simulink model "simulation"  (R2024b)
settings: Solver=ode45  StartTime=0.0  StopTime=10  MaxStep=0.001  RelTol=1e-2  AbsTol=1e-2  EnableMultiTasking=on
values from neighbouring files (symbols this model uses):
  m = subs(obj.M, [obj.theta0, obj.theta1, obj.theta2, obj.L], [a0, a1, a2, l])    [VMC_test.m]
  N = m_p*(x_ddot+L*theta_ddot*cos(theta)-L*theta_dot^2*sin(theta))+N_M    [LQR_wang.m]    (also in untitled.m = length(t))
  X = [x,x_dot,phi,phi_dot,theta,theta_dot].'    [LQR_wang.m]    (also in init.m = [x, d_x, phi, d_phi, theta, d_theta].'; raw.m = [x, d_x, phi, d_phi, theta, d_theta].')
undefined symbols (not defined in the file or in its folder): big_rod, little_rod, load, main_body, MO_L, motor, wheel, Y, Z
libraries: sm_lib x92, nesl_utility x49, slpidlib x2
(part 1 of 3)
settings Model: Creator=Orwell  LastModifiedBy=Orwell
settings SolverCC: AlgebraicLoopSolver=TrustRegion  MaxZcPerStep=1
settings DataIOCC: LimitDataPoints=on  MaxDataPoints=10000  ReturnWorkspaceOutputs=off
settings OptimizationCC: ReuseModelBlockBuffer=off  LifeSpan=inf
settings DebuggingCC: UnconnectedInputMsg=warning  UnconnectedOutputMsg=warning  UnconnectedLineMsg=warning  AllowSymbolicDim=off  SubsystemReferenceDiagnosticForUnitTest=warning  SFUnexpectedBacktrackingDiag=warning  SFNoUnconditionalDefaultTransitionDiag=warning  SFExecutionAtInitializationDiag=none  ArithmeticOperatorsInVariantConditions=warning
settings ModelReferenceCC: EnableRefExpFcnMdlSchedulingChecks=on
settings SFSimCC: SimUseLocalCustomCode=off  CustomCodeUndefinedFunction=UseInterfaceOnly
settings RTWCC: RTWUseLocalCustomCode=off  GPUComputeCapability=3.5  DLArmComputeVersion=19.05
settings CodeAppCC: StateflowObjectComments=on
settings GRTTargetCC: TargetLangStandard=C89/C90 (ANSI)
settings ConfigComp: CovMetricSettings=dw  CovSaveCumulativeToWorkspaceVar=on  CovSaveSingleToWorkspaceVar=on  CovExternalEMLEnable=off  CovSFcnEnable=off
settings SimscapeCC: SimscapeLogType=all  SimscapeLogSimulationStatistics=on  SimscapeLogDataHistory=10000

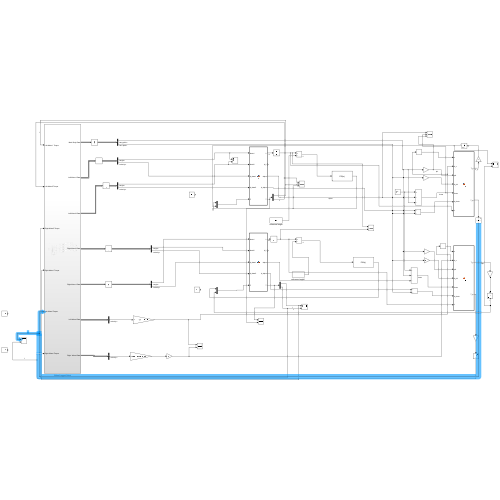
[thumbnail: Simulink's stored preview of the top-level diagram]
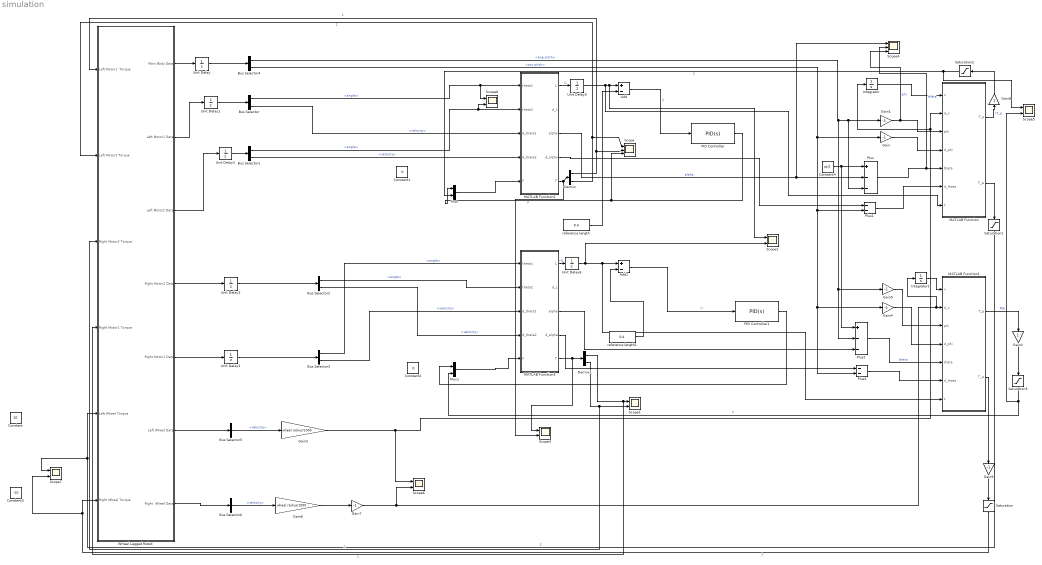
== system simulation ==
  Add : Sum  Inputs=+-
  Add1 : Sum  Inputs=+-
  Bus Selector{,1..3} (4 alike) : BusSelector  OutputSignals=angle,velocity
  Bus Selector4 : BusSelector  OutputSignals=ang pitch,acc pitch
  Bus Selector5 : BusSelector  OutputSignals=velocity
  Bus Selector6 : BusSelector  OutputSignals=velocity
  Constant : Constant  Value=10
  Constant1 : Constant  Value=0
  Constant2 : Constant  Value=0
  Constant3 : Constant  Value=-10
  Constant4 : Constant  Value=pi/2
  Demux : Demux  Outputs=2
  Demux1 : Demux  Outputs=2
  Gain{,1,4..5,7,9} (6 alike) : Gain  Gain=-1
  Gain2 : Gain  Gain=wheel.radius/1000
  Gain3 : Gain
  Gain6 : Gain  Gain=wheel.radius/1000
  Gain8 : Gain
  Integrator : Integrator
  Integrator1 : Integrator
  MATLAB Function : MATLAB Function  TreatAsAtomicUnit=on
  MATLAB Function1 : MATLAB Function  TreatAsAtomicUnit=on
  MATLAB Function2 : MATLAB Function  TreatAsAtomicUnit=on
  MATLAB Function3 : MATLAB Function  TreatAsAtomicUnit=on
  Mux : Mux  Inputs=2
  Mux1 : Mux  Inputs=2
  PID Controller : slpidlib/PID Controller  Controller=PID  Form=Parallel  TimeDomain=Continuous-time  UseExternalTs=off  SampleTime=-1  IntegratorMethod=Forward Euler  FilterMethod=Forward Euler  ControllerParametersSource=internal  P=2000  I=0  UseKiTs=off  D=0  UseExternalDerivativeSource=off  N=100  UseFilter=on  TunerSelectOption=Transfer Function Based (PID Tuner App)  InitialConditionSource=internal  InitialConditionForIntegrator=0  InitialConditionForFilter=0  DifferentiatorICPrevScaledInput=0  ExternalReset=none  TrackingMode=off  Kt=1  LimitOutput=off  SatLimitsSource=internal  UpperSaturationLimit=inf  LowerSaturationLimit=-inf  LinearizeAsGain=on  AntiWindupMode=none  Kb=1  LimitIntegrator=off  UpperIntegratorSaturationLimit=inf  LowerIntegratorSaturationLimit=-inf  POutMin=[]  POutMax=[]  IOutMin=[]  IOutMax=[]  DOutMin=[]  DOutMax=[]  NOutMin=[]  NOutMax=[]  SumOutMin=[]  SumOutMax=[]  SaturationOutMin=[]  SaturationOutMax=[]  PParamMin=[]  PParamMax=[]  IParamMin=[]  IParamMax=[]  DParamMin=[]  DParamMax=[]  NParamMin=[]  NParamMax=[]  KbParamMin=[]  KbParamMax=[]  KtParamMin=[]  KtParamMax=[]  KbOutMin=[]  KbOutMax=[]  KtOutMin=[]  KtOutMax=[]  IntegratorOutMin=[]  IntegratorOutMax=[]  FilterOutMin=[]  FilterOutMax=[]  SumI1OutMin=[]  SumI1OutMax=[]  SumI2OutMin=[]  SumI2OutMax=[]  SumI3OutMin=[]  SumI3OutMax=[]  SumI4OutMin=[]  SumI4OutMax=[]  SumDOutMin=[]  SumDOutMax=[]  DifferentiatorOutMin=[]  DifferentiatorOutMax=[]  FilterDiffOutCoefMin=[]  FilterDiffOutCoefMax=[]  ReciprocalOutMin=[]  ReciprocalOutMax=[]  SumDenOutMin=[]  SumDenOutMax=[]  SumNumOutMin=[]  SumNumOutMax=[]  DivideOutMin=[]  DivideOutMax=[]  UdiffTsProdOutMin=[]  UdiffTsProdOutMax=[]  NTsProdOutMin=[]  NTsProdOutMax=[]  UintegralTsProdOutMin=[]  UintegralTsProdOutMax=[]  UngainTsProdOutMin=[]  UngainTsProdOutMax=[]  ClampingZeroOutDataTypeStr=Inherit: Inherit via back propagation  ClampingZeroOutMin=[]  ClampingZeroOutMax=[]  FilterDenConstantOutDataTypeStr=Inherit: Inherit via back propagation  FilterDenConstantOutMin=[]  FilterDenConstantOutMax=[]  PCopyOutDataTypeStr=Inherit: Inherit via back propagation  PCopyOutMin=[]  PCopyOutMax=[]  NCopyOutDataTypeStr=Inherit: Inherit via back propagation  NCopyOutMin=[]  NCopyOutMax=[]  IntegratorContinuousStateAttributes=''  IntegratorStateMustResolveToSignalObject=off  IntegratorRTWStateStorageClass=Auto  FilterContinuousStateAttributes=''  FilterStateMustResolveToSignalObject=off  FilterRTWStateStorageClass=Auto  ParallelPVariant=InternalParameters  IdealPVariant=Disabled  IVariant=InternalParameters  DVariant=InternalParameters  IntegratorVariant=Continuous  SatVariant=Disabled  AWVariant=Passthrough  PCopyVariant=Disabled  TRVariant=Disabled  FdbkBlocksVariant=Forward  IdealPFdbkVariant=Disabled  SatFdbkVariant=Disabled  DerivativeFilterVariant=ContFilter  NVariant=InternalParameters  NCopyVariant=Disabled  FilterICVariant=InternalICsFilter  IntegratorICVariant=InternalICs  ExternalResetVariant=Disabled  TRSumVariant=Passthrough  SumFdbkVariant=Disabled  SumVariant=Sum_PID  TsampFilterVariant=InternalTs  TsampNgainVariant=Passthrough  TsampIntegralVariant=Disabled_SignalSpec  ExternalSaturationOutDataTypeStr=Inherit: Same as second input  DerivativeSourceVariant=ErrorSignal  PreIntVariant=InternalPreInt
  PID Controller1 : slpidlib/PID Controller  Controller=PID  Form=Parallel  TimeDomain=Continuous-time  UseExternalTs=off  SampleTime=-1  IntegratorMethod=Forward Euler  FilterMethod=Forward Euler  ControllerParametersSource=internal  P=2000  I=0  UseKiTs=off  D=0  UseExternalDerivativeSource=off  N=100  UseFilter=on  TunerSelectOption=Transfer Function Based (PID Tuner App)  InitialConditionSource=internal  InitialConditionForIntegrator=0  InitialConditionForFilter=0  DifferentiatorICPrevScaledInput=0  ExternalReset=none  TrackingMode=off  Kt=1  LimitOutput=off  SatLimitsSource=internal  UpperSaturationLimit=inf  LowerSaturationLimit=-inf  LinearizeAsGain=on  AntiWindupMode=none  Kb=1  LimitIntegrator=off  UpperIntegratorSaturationLimit=inf  LowerIntegratorSaturationLimit=-inf  POutMin=[]  POutMax=[]  IOutMin=[]  IOutMax=[]  DOutMin=[]  DOutMax=[]  NOutMin=[]  NOutMax=[]  SumOutMin=[]  SumOutMax=[]  SaturationOutMin=[]  SaturationOutMax=[]  PParamMin=[]  PParamMax=[]  IParamMin=[]  IParamMax=[]  DParamMin=[]  DParamMax=[]  NParamMin=[]  NParamMax=[]  KbParamMin=[]  KbParamMax=[]  KtParamMin=[]  KtParamMax=[]  KbOutMin=[]  KbOutMax=[]  KtOutMin=[]  KtOutMax=[]  IntegratorOutMin=[]  IntegratorOutMax=[]  FilterOutMin=[]  FilterOutMax=[]  SumI1OutMin=[]  SumI1OutMax=[]  SumI2OutMin=[]  SumI2OutMax=[]  SumI3OutMin=[]  SumI3OutMax=[]  SumI4OutMin=[]  SumI4OutMax=[]  SumDOutMin=[]  SumDOutMax=[]  DifferentiatorOutMin=[]  DifferentiatorOutMax=[]  FilterDiffOutCoefMin=[]  FilterDiffOutCoefMax=[]  ReciprocalOutMin=[]  ReciprocalOutMax=[]  SumDenOutMin=[]  SumDenOutMax=[]  SumNumOutMin=[]  SumNumOutMax=[]  DivideOutMin=[]  DivideOutMax=[]  UdiffTsProdOutMin=[]  UdiffTsProdOutMax=[]  NTsProdOutMin=[]  NTsProdOutMax=[]  UintegralTsProdOutMin=[]  UintegralTsProdOutMax=[]  UngainTsProdOutMin=[]  UngainTsProdOutMax=[]  ClampingZeroOutDataTypeStr=Inherit: Inherit via back propagation  ClampingZeroOutMin=[]  ClampingZeroOutMax=[]  FilterDenConstantOutDataTypeStr=Inherit: Inherit via back propagation  FilterDenConstantOutMin=[]  FilterDenConstantOutMax=[]  PCopyOutDataTypeStr=Inherit: Inherit via back propagation  PCopyOutMin=[]  PCopyOutMax=[]  NCopyOutDataTypeStr=Inherit: Inherit via back propagation  NCopyOutMin=[]  NCopyOutMax=[]  IntegratorContinuousStateAttributes=''  IntegratorStateMustResolveToSignalObject=off  IntegratorRTWStateStorageClass=Auto  FilterContinuousStateAttributes=''  FilterStateMustResolveToSignalObject=off  FilterRTWStateStorageClass=Auto  ParallelPVariant=InternalParameters  IdealPVariant=Disabled  IVariant=InternalParameters  DVariant=InternalParameters  IntegratorVariant=Continuous  SatVariant=Disabled  AWVariant=Passthrough  PCopyVariant=Disabled  TRVariant=Disabled  FdbkBlocksVariant=Forward  IdealPFdbkVariant=Disabled  SatFdbkVariant=Disabled  DerivativeFilterVariant=ContFilter  NVariant=InternalParameters  NCopyVariant=Disabled  FilterICVariant=InternalICsFilter  IntegratorICVariant=InternalICs  ExternalResetVariant=Disabled  TRSumVariant=Passthrough  SumFdbkVariant=Disabled  SumVariant=Sum_PID  TsampFilterVariant=InternalTs  TsampNgainVariant=Passthrough  TsampIntegralVariant=Disabled_SignalSpec  ExternalSaturationOutDataTypeStr=Inherit: Same as second input  DerivativeSourceVariant=ErrorSignal  PreIntVariant=InternalPreInt
  Plus : Sum  Inputs=+--
  Plus1 : Sum  Inputs=--
  Plus2 : Sum  Inputs=+--
  Plus3 : Sum  Inputs=--
  Saturation : Saturate  UpperLimit=1  LowerLimit=-1
  Saturation1 : Saturate  UpperLimit=1  LowerLimit=-1
  Saturation2 : Saturate  UpperLimit=500  LowerLimit=-500
  Saturation3 : Saturate  UpperLimit=500  LowerLimit=-500
  Scope : Scope  NumInputPorts=3
  Scope{1..3,5..8} (7 alike) : Scope  NumInputPorts=2
  Scope4 : Scope  NumInputPorts=3
  Unit Delay{,1..6} (7 alike) : UnitDelay  SampleTime=0.001  HasFrameUpgradeWarning=on
  WHeel Legged Robot : Subsystem
  reference length : Constant  Value=0.4
  reference length1 : Constant  Value=0.4
  wires:
  WHeel Legged Robot/2(Left Motor1 Data) -> Unit Delay1/1
  WHeel Legged Robot/3(Left Motor2 Data) -> Unit Delay2/1
  WHeel Legged Robot/4(Right Motor2 Data) -> Unit Delay3/1
  WHeel Legged Robot/5(Right Motor1 Data) -> Unit Delay4/1
  Bus Selector/1 -> Scope8/1, MATLAB Function2/1(theta1)  "<angle>"
  Bus Selector1/1 -> Scope8/2, MATLAB Function2/2(theta2)  "<angle>"
  Bus Selector/2 -> MATLAB Function2/3(d_theta1)  "<velocity>"
  Bus Selector1/2 -> MATLAB Function2/4(d_theta2)  "<velocity>"
  Mux/1 -> MATLAB Function2/5(F)
  MATLAB Function2/1(L) -> Unit Delay5/1  "Ll"
  reference length/1 -> Add/2
  PID Controller/1 -> Mux/1, Scope/3  "F"
  MATLAB Function2/5(T) -> Scope3/2, Demux/1
  Demux/1 -> WHeel Legged Robot/1(Left Motor1  Torque), Scope/2  "1"
  Demux/2 -> WHeel Legged Robot/2(Left Motor2 Torque), Scope/1  "2"
  PID Controller1/1 -> Mux1/1
  Mux1/1 -> MATLAB Function3/5(F)
  MATLAB Function3/1(L) -> Unit Delay6/1  "rlL"
  reference length1/1 -> Add1/2
  MATLAB Function3/5(T) -> Scope3/1, Demux1/1
  Demux1/1 -> WHeel Legged Robot/4(Right Motor1 Torque), Scope1/1  "1"
  Demux1/2 -> WHeel Legged Robot/3(RIght Motor2 Torque), Scope1/2  "2"
  Add/1 -> PID Controller/1  "ll"
  Add1/1 -> PID Controller1/1  "rl"
  Bus Selector2/2 -> MATLAB Function3/4(d_theta2)  "<velocity>"
  Bus Selector2/1 -> MATLAB Function3/2(theta2)  "<angle>"
  Bus Selector3/2 -> MATLAB Function3/3(d_theta1)  "<velocity>"
  Bus Selector3/1 -> MATLAB Function3/1(theta1)  "<angle>"
  WHeel Legged Robot/1(Main Body Data) -> Unit Delay/1
  Constant4/1 -> Plus2/1, Plus/1
  MATLAB Function2/3(alpha) -> Scope4/1, Plus/2  "alpha"
  Bus Selector4/1 -> Gain5/1, Plus2/2, Gain1/1, Plus/3  "<ang pitch>"
  Plus/1 -> Scope4/2, MATLAB Function/5(theta)  "theta"
  Plus1/1 -> MATLAB Function/6(d_theta)
  MATLAB Function2/4(d_alpha) -> Plus1/1
  Bus Selector4/2 -> Plus3/2, Gain4/1, Plus1/2, Gain/1  "<acc pitch>"
  Gain/1 -> MATLAB Function/4(d_phi)
  Gain1/1 -> Scope4/3, MATLAB Function/3(phi)  "phi"
  WHeel Legged Robot/6(Left Wheel Data) -> Bus Selector5/1
  Bus Selector5/1 -> Gain2/1  "<velocity>"
  Gain2/1 -> Scope6/1, Integrator/1, MATLAB Function/2(d_x)
  Integrator/1 -> MATLAB Function/1(x)
  Unit Delay/1 -> Bus Selector4/1
  Unit Delay1/1 -> Bus Selector/1
  Unit Delay2/1 -> Bus Selector1/1
  Unit Delay3/1 -> Bus Selector2/1
  Unit Delay4/1 -> Bus Selector3/1
  Unit Delay5/1 -> MATLAB Function/7(L), Scope2/1, Add/1
  MATLAB Function/1(T_p) -> Gain8/1  "lT_p"
  MATLAB Function1/1(T_p) -> Gain3/1  "Rtp"
  MATLAB Function1/2(T_w) -> Gain9/1
  Gain4/1 -> MATLAB Function1/4(d_phi)
  Plus3/1 -> MATLAB Function1/6(d_theta)
  MATLAB Function3/4(d_alpha) -> Plus3/1
  Plus2/1 -> MATLAB Function1/5(theta)  "theta"
  Gain5/1 -> MATLAB Function1/3(phi)
  MATLAB Function3/3(alpha) -> Plus2/3
  WHeel Legged Robot/7(Right  Wheel Data) -> Bus Selector6/1
  Bus Selector6/1 -> Gain6/1  "<velocity>"
  Gain6/1 -> Gain7/1
  Gain7/1 -> Scope6/2, Integrator1/1, MATLAB Function1/2(d_x)
  Integrator1/1 -> MATLAB Function1/1(x)
  Unit Delay6/1 -> Scope2/2, MATLAB Function1/7(L), Add1/1
  Saturation/1 -> WHeel Legged Robot/6(Right Wheel Torque), Scope7/2  "1"
  Saturation1/1 -> WHeel Legged Robot/5(Left Wheel Torque), Scope7/1  "2"
  MATLAB Function/2(T_w) -> Saturation1/1
  Saturation2/1 -> Scope5/1, Mux/2  "2"
  Saturation3/1 -> Mux1/2, Scope5/2  "2"
  Gain3/1 -> Saturation3/1
  Gain8/1 -> Saturation2/1
  Gain9/1 -> Saturation/1

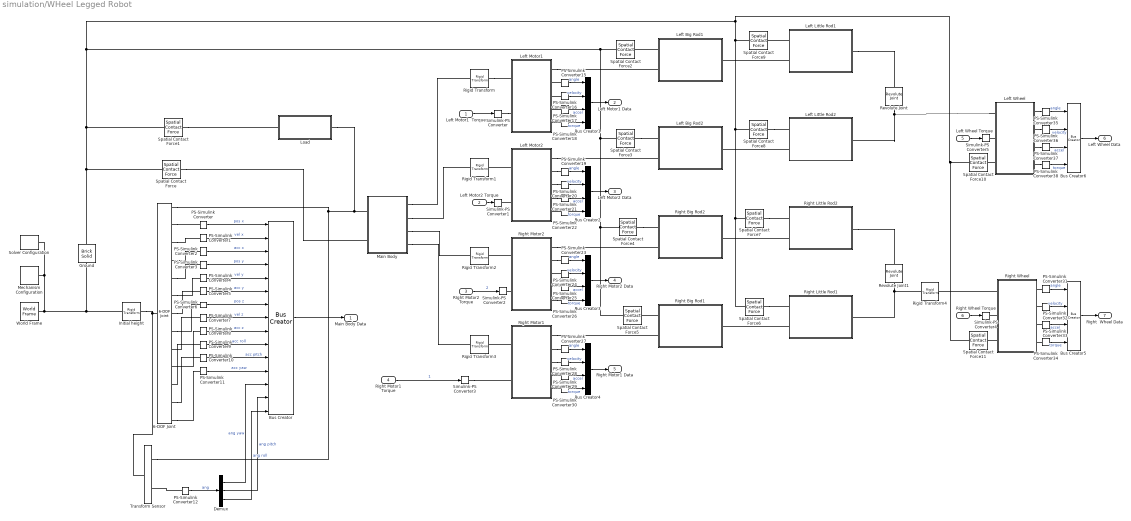
== system simulation/WHeel Legged Robot ==
  Left Motor1  Torque : Inport
  Left Motor2 Torque : Inport  Port=2
  RIght Motor2 Torque : Inport  Port=3
  Right Motor1 Torque : Inport  Port=4
  Left Wheel Torque : Inport  Port=5
  Right Wheel Torque : Inport  Port=6
  6-DOF Joint : sm_lib/Joints/6-DOF Joint  JointMode=Normal  CompositeWrenchDir=FollowerOnBase  CompositeWrenchFrame=BaseFrame  SenseConstraintForce=off  SenseConstraintTorque=off  SenseTotalForce=off  SenseTotalTorque=off  PxPositionTargetSpecify=off  PxPositionTargetPriority=High  PxPositionTargetValue=0  PxPositionTargetValueUnits=m  PxVelocityTargetSpecify=off  PxVelocityTargetPriority=High  PxVelocityTargetValue=0  PxVelocityTargetValueUnits=m/s  PxEquilibriumPosition=0  PxEquilibriumPositionUnits=m  PxSpringStiffness=0  PxSpringStiffnessUnits=N/m  PxDampingCoefficient=0  PxDampingCoefficientUnits=N/(m/s)  PxLowerLimitSpecify=off  PxLowerLimitBound=-1  PxLowerLimitBoundUnits=m  PxLowerLimitStiffness=1e6  PxLowerLimitStiffnessUnits=N/m  PxLowerLimitDamping=1e3  PxLowerLimitDampingUnits=N/(m/s)  PxLowerLimitTransitionRegionWidth=1e-4  PxLowerLimitTransitionRegionWidthUnits=m  PxUpperLimitSpecify=off  PxUpperLimitBound=1  PxUpperLimitBoundUnits=m  PxUpperLimitStiffness=1e6  PxUpperLimitStiffnessUnits=N/m  PxUpperLimitDamping=1e3  PxUpperLimitDampingUnits=N/(m/s)  PxUpperLimitTransitionRegionWidth=1e-4  PxUpperLimitTransitionRegionWidthUnits=m  PxTorqueActuationMode=NoTorque  PxMotionActuationMode=ComputedMotion  PxSensePosition=on  PxSenseVelocity=on  PxSenseAcceleration=on  PxSenseTorqueForce=off  PxSenseLowerLimitTorqueForce=off  PxSenseUpperLimitTorqueForce=off  PyPositionTargetSpecify=off  PyPositionTargetPriority=High  PyPositionTargetValue=0  PyPositionTargetValueUnits=m  PyVelocityTargetSpecify=off  PyVelocityTargetPriority=High  PyVelocityTargetValue=0  PyVelocityTargetValueUnits=m/s  PyEquilibriumPosition=0  PyEquilibriumPositionUnits=m  PySpringStiffness=0  PySpringStiffnessUnits=N/m  PyDampingCoefficient=0  PyDampingCoefficientUnits=N/(m/s)  PyLowerLimitSpecify=off  PyLowerLimitBound=-1  PyLowerLimitBoundUnits=m  PyLowerLimitStiffness=1e6  PyLowerLimitStiffnessUnits=N/m  PyLowerLimitDamping=1e3  PyLowerLimitDampingUnits=N/(m/s)  PyLowerLimitTransitionRegionWidth=1e-4  PyLowerLimitTransitionRegionWidthUnits=m  PyUpperLimitSpecify=off  PyUpperLimitBound=1  PyUpperLimitBoundUnits=m  PyUpperLimitStiffness=1e6  PyUpperLimitStiffnessUnits=N/m  PyUpperLimitDamping=1e3  PyUpperLimitDampingUnits=N/(m/s)  PyUpperLimitTransitionRegionWidth=1e-4  PyUpperLimitTransitionRegionWidthUnits=m  PyTorqueActuationMode=NoTorque  PyMotionActuationMode=ComputedMotion  PySensePosition=on  PySenseVelocity=on  PySenseAcceleration=on  PySenseTorqueForce=off  PySenseLowerLimitTorqueForce=off  PySenseUpperLimitTorqueForce=off  PzPositionTargetSpecify=off  PzPositionTargetPriority=High  PzPositionTargetValue=0  PzPositionTargetValueUnits=m  PzVelocityTargetSpecify=off  PzVelocityTargetPriority=High  PzVelocityTargetValue=0  PzVelocityTargetValueUnits=m/s  PzEquilibriumPosition=0  PzEquilibriumPositionUnits=m  PzSpringStiffness=0  PzSpringStiffnessUnits=N/m  PzDampingCoefficient=0  PzDampingCoefficientUnits=N/(m/s)  PzLowerLimitSpecify=off  PzLowerLimitBound=-1  PzLowerLimitBoundUnits=m  PzLowerLimitStiffness=1e6  PzLowerLimitStiffnessUnits=N/m  PzLowerLimitDamping=1e3  PzLowerLimitDampingUnits=N/(m/s)  PzLowerLimitTransitionRegionWidth=1e-4  PzLowerLimitTransitionRegionWidthUnits=m  PzUpperLimitSpecify=off  PzUpperLimitBound=1  PzUpperLimitBoundUnits=m  PzUpperLimitStiffness=1e6  PzUpperLimitStiffnessUnits=N/m  PzUpperLimitDamping=1e3  PzUpperLimitDampingUnits=N/(m/s)  PzUpperLimitTransitionRegionWidth=1e-4  PzUpperLimitTransitionRegionWidthUnits=m  PzTorqueActuationMode=NoTorque  PzMotionActuationMode=ComputedMotion  PzSensePosition=on  PzSenseVelocity=on  PzSenseAcceleration=on  PzSenseTorqueForce=off  PzSenseLowerLimitTorqueForce=off  PzSenseUpperLimitTorqueForce=off  SphPositionTargetSpecify=off  SphPositionTargetPriority=High  SphPositionTargetRotationMethod=StandardAxis  SphPositionTargetFollAlignAxisA=+X  SphPositionTargetBaseAlignAxisA=+Y  SphPositionTargetFollAlignAxisB=+Y  SphPositionTargetBaseAlignAxisB=+Z  SphPositionTargetRotationStandardAxis=+Y  SphPositionTargetRotationAngle=90  SphPositionTargetRotationAngleUnits=deg  SphPositionTargetRotationArbitraryAxis=[0 0 1]  SphPositionTargetRotationSequenceAxes=FollowerAxes  SphPositionTargetRotationSequence=XYX  SphPositionTargetRotationSequenceAngles=[0 0 0]  SphPositionTargetRotationSequenceAnglesUnits=deg  SphPositionTargetRotationMatrix=[1 0 0;0 1 0;0 0 1]  SphPositionTargetQuaternion=[1 0 0 0]  SphVelocityTargetSpecify=off  SphVelocityTargetPriority=High  SphVelocityTargetValue=[0 0 0]  SphVelocityTargetValueUnits=deg/s  SphVelocityTargetInFollowerFrame=on  SphEqPosRotationMethod=None  SphEqPosFollAlignAxisA=+X  SphEqPosBaseAlignAxisA=+Y  SphEqPosFollAlignAxisB=+Y  SphEqPosBaseAlignAxisB=+Z  SphEqPosRotationStandardAxis=+Z  SphEqPosRotationAngle=0  SphEqPosRotationAngleUnits=deg  SphEqPosRotationArbitraryAxis=[0 0 1]  SphEqPosRotationSequenceAxes=FollowerAxes  SphEqPosRotationSequence=XYX  SphEqPosRotationSequenceAngles=[0 0 0]  SphEqPosRotationSequenceAnglesUnits=deg  SphEqPosRotationMatrix=[1 0 0;0 1 0;0 0 1]  SphEqPosQuaternion=[1 0 0 0]  SphSpringStiffness=0  SphSpringStiffnessUnits=N*m/deg  SphDampingCoefficient=0  SphDampingCoefficientUnits=N*m/(deg/s)  SphLowerLimitSpecify=off  SphLowerLimitBound=15  SphLowerLimitBoundUnits=deg  SphLowerLimitStiffness=1e4  SphLowerLimitStiffnessUnits=N*m/deg  SphLowerLimitDamping=10  SphLowerLimitDampingUnits=N*m/(deg/s)  SphLowerLimitTransitionRegionWidth=0.1  SphLowerLimitTransitionRegionWidthUnits=deg  SphUpperLimitSpecify=off  SphUpperLimitBound=45  SphUpperLimitBoundUnits=deg  SphUpperLimitStiffness=1e4  SphUpperLimitStiffnessUnits=N*m/deg  SphUpperLimitDamping=10  SphUpperLimitDampingUnits=N*m/(deg/s)  SphUpperLimitTransitionRegionWidth=0.1  SphUpperLimitTransitionRegionWidthUnits=deg  SphTorqueActuationMode=NoTorque  SphActuateTorqueX=off  SphActuateTorqueY=off  SphActuateTorqueZ=off  SphActuateTorque=off  SphActuationFrame=BaseFrame  SphSensePosition=off  SphSenseVelocityX=on  SphSenseVelocityY=on  SphSenseVelocityZ=on  SphSenseVelocity=off  SphSenseAccelerationX=off  SphSenseAccelerationY=off  SphSenseAccelerationZ=off  SphSenseAcceleration=off  SphSenseLowerLimitTorqueMag=off  SphSenseUpperLimitTorqueMag=off  SphSensingFrame=BaseFrame
  Bus Creator : BusCreator  Inputs=15
  Bus Creator{1..6} (6 alike) : BusCreator  Inputs=4
  Demux : Demux  Outputs=3
  Ground : sm_lib/Body Elements/Brick Solid  BrickDimensions=[6 2 0.2]  BrickDimensionsUnits=m  ExportEntireGeometry=on  InertiaType=CalculateFromGeometry  BasedOnType=Density  Density=1000  DensityUnits=kg/m^3  Mass=1  MassUnits=kg  CenterOfMass=[0 0 0]  CenterOfMassUnits=m  MomentsOfInertia=[1 1 1]  MomentsOfInertiaUnits=kg*m^2  ProductsOfInertia=[0 0 0]  ProductsOfInertiaUnits=kg*m^2  GraphicType=FromGeometry  MarkerShape=Sphere  MarkerSize=10  GraphicVisPropType=SimpleVisualProperties  GraphicDiffuseColor=[0 0 0]  GraphicOpacity=1  GraphicSpecularColor=[0.5 0.5 0.5 1.0]  GraphicAmbientColor=[0.15 0.15 0.15 1.0]  GraphicEmissiveColor=[0.0 0.0 0.0 1.0]  GraphicShininess=75  DoExposeReferenceFrame=on  SerializedFrames=<Frames/>
  Initial height : sm_lib/Frames and Transforms/Rigid Transform  RotationMethod=None  FollAlignAxisA=+X  BaseAlignAxisA=+Y  FollAlignAxisB=+Y  BaseAlignAxisB=+Z  RotationStandardAxis=+Z  RotationAngle=0  RotationAngleUnits=deg  RotationArbitraryAxis=[0 0 1]  RotationSequenceAxes=FollowerAxes  RotationSequence=XYX  RotationSequenceAngles=[0 0 0]  RotationSequenceAnglesUnits=deg  RotationMatrix=[1 0 0;0 1 0;0 0 1]  Quaternion=[1 0 0 0]  TranslationMethod=StandardAxis  TranslationCartesianOffset=[0 0 0]  TranslationCartesianOffsetUnits=m  TranslationStandardAxis=+Z  TranslationStandardOffset=initial_height  TranslationStandardOffsetUnits=mm  TranslationROffset=0  TranslationROffsetUnits=m  TranslationThetaOffset=0  TranslationThetaOffsetUnits=deg  TranslationZOffset=0  TranslationZOffsetUnits=m
  Left Big Rod1 : Subsystem  mask{BR_L=big_rod.length, BR_W=big_rod.width, BR_H=big_rod.height, BR_M=big_rod.mass, JO_Max_A=0, JO_Min_A=0}
      mask prompts: BR_L "Big Rod Length"; BR_W "BIg Rod Width"; BR_H "Big Rod Height"; BR_M "Big Rod Mass"; JO_Max_A "Joint Max Angle"; JO_Min_A "Joint Min Angle"
      mask DialogControl ParameterGroupVar Prompt: 参数
  Left Big Rod2 : Subsystem  mask{BR_L=big_rod.length, BR_W=big_rod.width, BR_H=big_rod.height, BR_M=big_rod.mass}
      mask prompts: BR_L "Big Rod Length"; BR_W "BIg Rod Width"; BR_H "Big Rod Height"; BR_M "Big Rod Mass"
      mask DialogControl ParameterGroupVar Prompt: 参数
  Left Little Rod1 : Subsystem  mask{LR_L=little_rod.length, LR_W=little_rod.width, LR_H=little_rod.height, LR_M=little_rod.mass}
      mask prompts: LR_L "Little Rod Length"; LR_W "LittleRod Width"; LR_H "Little Rod Height"; LR_M "Little Rod Mass"
      mask DialogControl ParameterGroupVar Prompt: 参数
  Left Little Rod2 : Subsystem  mask{LR_L=little_rod.length, LR_W=little_rod.width, LR_H=little_rod.height, LR_M=little_rod.mass}
      mask prompts: LR_L "Little Rod Length"; LR_W "LittleRod Width"; LR_H "Little Rod Height"; LR_M "Little Rod Mass"
      mask DialogControl ParameterGroupVar Prompt: 参数
  Left Motor1 : Subsystem  mask{MO_R=motor.radius, MO_L=motor.length, MO_M=motor.mass, MO_Max_A=50, MO_Min_A=-12}
      mask prompts: MO_R "Motor Radius"; MO_L "Motor Length"; MO_M "Motor Mass"; MO_Max_A "Motor Max Angle"; MO_Min_A "Motor Mini Angle"
      mask DialogControl ParameterGroupVar Prompt: 参数
  Left Motor2 : Subsystem  mask{MO_R=motor.radius, MO_L=motor.length, MO_M=motor.mass, MO_Max_A=192, MO_Min_A=110}
      mask prompts: MO_R "Motor Radius"; MO_L "Motor Length"; MO_M "Motor Mass"; MO_Max_A "Motor Max Angle"; MO_Min_A "Motor Mini Angle"
      mask DialogControl ParameterGroupVar Prompt: 参数
  Left Wheel : Subsystem  mask{WO_R=wheel.radius, WO_L=wheel.length, WO_M=wheel.mass}
      mask prompts: WO_R "Wheel Radius"; WO_L "Wheel Length"; WO_M "Wheel Mass"
      mask DialogControl ParameterGroupVar Prompt: 参数
  Load : Subsystem  mask{LO_L=load.length, LO_W=load.width, LO_H=load.hight, LO_M=load.mass}
      mask prompts: LO_L "Load Length"; LO_W "Load Width"; LO_H "Load Height"; LO_M "Load Mass"
      mask DialogControl ParameterGroupVar Prompt: 参数
  Main Body : Subsystem  mask{LM1_PosX=motor.postion_x, LM1_PosY=motor.postion_y, LM2_PosX=motor.postion_x, LM2_PosY=motor.postion_y, RM1_PosX=motor.postion_x, RM1_PosY=motor.postion_y, RM2_PosX=motor.postion_x, RM2_PosY=motor.postion_y, Load_Pos=load.position_y, MB_L=main_body.length, MB_W=main_body.width, MB_H=main_body.hight, MB_M=main_body.mass}
      mask prompts: LM1_PosX "Left Motor1 Position X"; LM1_PosY "Left Motor1 Position Y"; LM2_PosX "Left Motor2 Position X"; LM2_PosY "Left Motor2 Position Y"; RM1_PosX "Right Motor1 Position X"; RM1_PosY "Right Motor1 Position Y"; RM2_PosX "Right Motor2 Position X"; RM2_PosY "Right Motor2 Position Y"; Load_Pos "Load Position Y"; MB_L "Main Body Length"; MB_W "Main Body Width"; MB_H "Main Body Hight"; MB_M "Main Body Mass"
      mask DialogControl ParameterGroupVar Prompt: 参数
  Mechanism Configuration : sm_lib/Utilities/Mechanism Configuration  UniformGravity=Constant  GravityVector="[0  0 -9.80665 ]"  GravityVectorUnits=m/s^2  LinearizationDelta=0.001  JointModeTransitionNonlinearIterations=2
  PS-Simulink Converter{,1..12,15..38} (37 alike) : nesl_utility/PS-Simulink Converter  PhysicalDomain=network_engine_domain  SubClassName=ps_output  LeftPortType=input  RightPortType=output  PseudoPeriodic=off  Frequencies=[]  VectorFormat=inherit  Unit=inherit  AffineConversion=off
  Revolute Joint : sm_lib/Joints/Revolute Joint  JointMode=Normal  CompositeWrenchDir=FollowerOnBase  CompositeWrenchFrame=BaseFrame  SenseConstraintForce=off  SenseConstraintTorque=off  SenseTotalForce=off  SenseTotalTorque=off  PositionTargetSpecify=off  PositionTargetPriority=High  PositionTargetValue=0  PositionTargetValueUnits=deg  VelocityTargetSpecify=off  VelocityTargetPriority=High  VelocityTargetValue=0  VelocityTargetValueUnits=deg/s  EquilibriumPosition=0  EquilibriumPositionUnits=deg  SpringStiffness=0  SpringStiffnessUnits=N*m/deg  DampingCoefficient=0  DampingCoefficientUnits=N*m/(deg/s)  LowerLimitSpecify=off  LowerLimitBound=-90  LowerLimitBoundUnits=deg  LowerLimitStiffness=1e4  LowerLimitStiffnessUnits=N*m/deg  LowerLimitDamping=10  LowerLimitDampingUnits=N*m/(deg/s)  LowerLimitTransitionRegionWidth=0.1  LowerLimitTransitionRegionWidthUnits=deg  UpperLimitSpecify=off  UpperLimitBound=90  UpperLimitBoundUnits=deg  UpperLimitStiffness=1e4  UpperLimitStiffnessUnits=N*m/deg  UpperLimitDamping=10  UpperLimitDampingUnits=N*m/(deg/s)  UpperLimitTransitionRegionWidth=0.1  UpperLimitTransitionRegionWidthUnits=deg  TorqueActuationMode=NoTorque  MotionActuationMode=ComputedMotion  SensePosition=off  SenseVelocity=off  SenseAcceleration=off  SenseTorqueForce=off  SenseLowerLimitTorqueForce=off  SenseUpperLimitTorqueForce=off
  Revolute Joint1 : sm_lib/Joints/Revolute Joint  JointMode=Normal  CompositeWrenchDir=FollowerOnBase  CompositeWrenchFrame=BaseFrame  SenseConstraintForce=off  SenseConstraintTorque=off  SenseTotalForce=off  SenseTotalTorque=off  PositionTargetSpecify=off  PositionTargetPriority=High  PositionTargetValue=0  PositionTargetValueUnits=deg  VelocityTargetSpecify=off  VelocityTargetPriority=High  VelocityTargetValue=0  VelocityTargetValueUnits=deg/s  EquilibriumPosition=0  EquilibriumPositionUnits=deg  SpringStiffness=0  SpringStiffnessUnits=N*m/deg  DampingCoefficient=0  DampingCoefficientUnits=N*m/(deg/s)  LowerLimitSpecify=off  LowerLimitBound=-90  LowerLimitBoundUnits=deg  LowerLimitStiffness=1e4  LowerLimitStiffnessUnits=N*m/deg  LowerLimitDamping=10  LowerLimitDampingUnits=N*m/(deg/s)  LowerLimitTransitionRegionWidth=0.1  LowerLimitTransitionRegionWidthUnits=deg  UpperLimitSpecify=off  UpperLimitBound=90  UpperLimitBoundUnits=deg  UpperLimitStiffness=1e4  UpperLimitStiffnessUnits=N*m/deg  UpperLimitDamping=10  UpperLimitDampingUnits=N*m/(deg/s)  UpperLimitTransitionRegionWidth=0.1  UpperLimitTransitionRegionWidthUnits=deg  TorqueActuationMode=NoTorque  MotionActuationMode=ComputedMotion  SensePosition=off  SenseVelocity=off  SenseAcceleration=off  SenseTorqueForce=off  SenseLowerLimitTorqueForce=off  SenseUpperLimitTorqueForce=off
  Right Big Rod1 : Subsystem  mask{BR_L=big_rod.length, BR_W=big_rod.width, BR_H=big_rod.height, BR_M=big_rod.mass}
      mask prompts: BR_L "Big Rod Length"; BR_W "BIg Rod Width"; BR_H "Big Rod Height"; BR_M "Big Rod Mass"
      mask DialogControl ParameterGroupVar Prompt: 参数
  Right Big Rod2 : Subsystem  mask{BR_L=big_rod.length, BR_W=big_rod.width, BR_H=big_rod.height, BR_M=big_rod.mass}
      mask prompts: BR_L "Big Rod Length"; BR_W "BIg Rod Width"; BR_H "Big Rod Height"; BR_M "Big Rod Mass"
      mask DialogControl ParameterGroupVar Prompt: 参数
  Right Little Rod1 : Subsystem  mask{LR_L=little_rod.length, LR_W=little_rod.width, LR_H=little_rod.height, LR_M=little_rod.mass}
      mask prompts: LR_L "Little Rod Length"; LR_W "LittleRod Width"; LR_H "Little Rod Height"; LR_M "Little Rod Mass"
      mask DialogControl ParameterGroupVar Prompt: 参数
  Right Little Rod2 : Subsystem  mask{LR_L=little_rod.length, LR_W=little_rod.width, LR_H=little_rod.height, LR_M=little_rod.mass}
      mask prompts: LR_L "Little Rod Length"; LR_W "LittleRod Width"; LR_H "Little Rod Height"; LR_M "Little Rod Mass"
      mask DialogControl ParameterGroupVar Prompt: 参数
  Right Motor1 : Subsystem  mask{MO_R=motor.radius, MO_L=motor.length, MO_M=motor.mass, MO_Max_A=50, MO_Min_A=-12}
      mask prompts: MO_R "Motor Radius"; MO_L "Motor Length"; MO_M "Motor Mass"; MO_Max_A "Motor Max Angle"; MO_Min_A "Motor Mini Angle"
      mask DialogControl ParameterGroupVar Prompt: 参数
  Right Motor2 : Subsystem  mask{MO_R=motor.radius, MO_L=motor.length, MO_M=motor.mass, MO_Max_A=192, MO_Min_A=110}
      mask prompts: MO_R "Motor Radius"; MO_L "Motor Length"; MO_M "Motor Mass"; MO_Max_A "Motor Max Angle"; MO_Min_A "Motor Mini Angle"
      mask DialogControl ParameterGroupVar Prompt: 参数
  Right Wheel : Subsystem  mask{WO_R=wheel.radius, WO_L=wheel.length, WO_M=wheel.mass}
      mask prompts: WO_R "Wheel Radius"; WO_L "Wheel Length"; WO_M "Wheel Mass"
      mask DialogControl ParameterGroupVar Prompt: 参数
  Rigid Transform : sm_lib/Frames and Transforms/Rigid Transform  RotationMethod=StandardAxis  FollAlignAxisA=+X  BaseAlignAxisA=+Y  FollAlignAxisB=+Y  BaseAlignAxisB=+Z  RotationStandardAxis=+X  RotationAngle=90  RotationAngleUnits=deg  RotationArbitraryAxis=[0 0 1]  RotationSequenceAxes=FollowerAxes  RotationSequence=XYX  RotationSequenceAngles=[0 0 0]  RotationSequenceAnglesUnits=deg  RotationMatrix=[1 0 0;0 1 0;0 0 1]  Quaternion=[1 0 0 0]  TranslationMethod=None  TranslationCartesianOffset=[0 0 0]  TranslationCartesianOffsetUnits=m  TranslationStandardAxis=+Z  TranslationStandardOffset=0  TranslationStandardOffsetUnits=m  TranslationROffset=0  TranslationROffsetUnits=m  TranslationThetaOffset=0  TranslationThetaOffsetUnits=deg  TranslationZOffset=0  TranslationZOffsetUnits=m
  Rigid Transform1 : sm_lib/Frames and Transforms/Rigid Transform  RotationMethod=StandardAxis  FollAlignAxisA=+X  BaseAlignAxisA=+Y  FollAlignAxisB=+Y  BaseAlignAxisB=+Z  RotationStandardAxis=+X  RotationAngle=90  RotationAngleUnits=deg  RotationArbitraryAxis=[0 0 1]  RotationSequenceAxes=FollowerAxes  RotationSequence=XYX  RotationSequenceAngles=[0 0 0]  RotationSequenceAnglesUnits=deg  RotationMatrix=[1 0 0;0 1 0;0 0 1]  Quaternion=[1 0 0 0]  TranslationMethod=None  TranslationCartesianOffset=[0 0 0]  TranslationCartesianOffsetUnits=m  TranslationStandardAxis=+Z  TranslationStandardOffset=0  TranslationStandardOffsetUnits=m  TranslationROffset=0  TranslationROffsetUnits=m  TranslationThetaOffset=0  TranslationThetaOffsetUnits=deg  TranslationZOffset=0  TranslationZOffsetUnits=m
  Rigid Transform2 : sm_lib/Frames and Transforms/Rigid Transform  RotationMethod=StandardAxis  FollAlignAxisA=+X  BaseAlignAxisA=+Y  FollAlignAxisB=+Y  BaseAlignAxisB=+Z  RotationStandardAxis=-X  RotationAngle=90  RotationAngleUnits=deg  RotationArbitraryAxis=[0 0 1]  RotationSequenceAxes=FollowerAxes  RotationSequence=XYX  RotationSequenceAngles=[0 0 0]  RotationSequenceAnglesUnits=deg  RotationMatrix=[1 0 0;0 1 0;0 0 1]  Quaternion=[1 0 0 0]  TranslationMethod=None  TranslationCartesianOffset=[0 0 0]  TranslationCartesianOffsetUnits=m  TranslationStandardAxis=+Z  TranslationStandardOffset=0  TranslationStandardOffsetUnits=m  TranslationROffset=0  TranslationROffsetUnits=m  TranslationThetaOffset=0  TranslationThetaOffsetUnits=deg  TranslationZOffset=0  TranslationZOffsetUnits=m
  Rigid Transform3 : sm_lib/Frames and Transforms/Rigid Transform  RotationMethod=StandardAxis  FollAlignAxisA=+X  BaseAlignAxisA=+Y  FollAlignAxisB=+Y  BaseAlignAxisB=+Z  RotationStandardAxis=-X  RotationAngle=90  RotationAngleUnits=deg  RotationArbitraryAxis=[0 0 1]  RotationSequenceAxes=FollowerAxes  RotationSequence=XYX  RotationSequenceAngles=[0 0 0]  RotationSequenceAnglesUnits=deg  RotationMatrix=[1 0 0;0 1 0;0 0 1]  Quaternion=[1 0 0 0]  TranslationMethod=None  TranslationCartesianOffset=[0 0 0]  TranslationCartesianOffsetUnits=m  TranslationStandardAxis=+Z  TranslationStandardOffset=0  TranslationStandardOffsetUnits=m  TranslationROffset=0  TranslationROffsetUnits=m  TranslationThetaOffset=0  TranslationThetaOffsetUnits=deg  TranslationZOffset=0  TranslationZOffsetUnits=m
  Rigid Transform4 : sm_lib/Frames and Transforms/Rigid Transform  RotationMethod=StandardAxis  FollAlignAxisA=+X  BaseAlignAxisA=+Y  FollAlignAxisB=+Y  BaseAlignAxisB=+Z  RotationStandardAxis=+X  RotationAngle=180  RotationAngleUnits=deg  RotationArbitraryAxis=[0 0 1]  RotationSequenceAxes=FollowerAxes  RotationSequence=XYX  RotationSequenceAngles=[0 0 0]  RotationSequenceAnglesUnits=deg  RotationMatrix=[1 0 0;0 1 0;0 0 1]  Quaternion=[1 0 0 0]  TranslationMethod=None  TranslationCartesianOffset=[0 0 0]  TranslationCartesianOffsetUnits=m  TranslationStandardAxis=-Z  TranslationStandardOffset=MO_L/2  TranslationStandardOffsetUnits=mm  TranslationROffset=0  TranslationROffsetUnits=m  TranslationThetaOffset=0  TranslationThetaOffsetUnits=deg  TranslationZOffset=0  TranslationZOffsetUnits=m
  Simulink-PS Converter{,1..5} (6 alike) : nesl_utility/Simulink-PS Converter  PhysicalDomain=network_engine_domain  SubClassName=ps_input  LeftPortType=input  RightPortType=output  PseudoPeriodic=off  Frequencies=[]  NoiseDistribution=none  NoiseParameters=[]  Unit=1  AffineConversion=off  FilteringAndDerivatives=provide  SimscapeFilterOrder=1  InputFilterTimeConstant=0.001  UdotUserProvided=0
  Solver Configuration : nesl_utility/Solver Configuration  PhysicalDomain=network_engine_domain  SubClassName=solver  LeftPortType=input  RightPortType=generic  Tones=[]  Harmonics=[]  SimulateNoise=off  Profile=off  UseLocalSampling=off  EnableSwitchedLinearOptims=on  FrequencyDomain=off  UseCCode=off  RelTol=0.001  AbsTol=1e-06  MinStep=1e-09  ToWorkspace=off  RevertToSquareIcSolve=off  NumHomotopyIterations=100  PhasorMode=off  PhasorModeNumHarmonics=1  ConsistencySolver=NEWTON_XTOL_AFTER_FTOL  IndexReductionMethod=DerivativeReplacement  DoDC=off  ResidualTolerance=1e-09  ConsistencyTolSource=GLOBAL  ConsistencyAbsTol=0.001  ConsistencyRelTol=0.001  ConsistencyTolFactor=0.001  UseLocalSolver=off  LocalSolverChoice=NE_BACKWARD_EULER_ADVANCER  ResolveIndetEquations=on  FunctionEvalNumThread=1  LocalSolverSampleTime=0.001  DoFixedCost=off  MaxNonlinIter=3  MaxModeIter=2  ComputeImpulses=off  ImpulseIterations=2  LinearAlgebra=Sparse  LinearAlgebraNumThread=0  EquationFormulation=NE_TIME_EF  DelaysMemoryBudget=1024  AutomaticFiltering=on  FilteringTimeConstant=0.001  PartitionStorageMethod=AS_NEEDED  PartitionMemoryBudget=1024  PartitionMethod=FAST  MultibodyUseLocalSolver=off  MultibodyLocalSolverChoice=ODE1  MultibodyLocalSolverSampleTime=0.001
  Spatial Contact Force{,1..11} (12 alike) : sm_lib/Forces and Torques/Spatial Contact Force  NormalForceType=SmoothSpringDamper  NormalStiffness=1e6  NormalStiffnessUnits=N/m  NormalDamping=1e3  NormalDampingUnits=N/(m/s)  NormalTransitionRegionWidth=1e-4  NormalTransitionRegionWidthUnits=m  FrictionType=SmoothStickSlip  CoefficientOfStaticFriction=0.5  CoefficientOfDynamicFriction=0.3  FrictionalCriticalVelocity=1e-3  FrictionalCriticalVelocityUnits=m/s  SenseContactSignal=off  SensePenetrationDepth=off  SenseSeparationDistance=off  SenseNormalForceMagnitude=off  SenseFrictionalForceMagnitude=off  SenseNormalVelocity=off  SenseTangentialVelocity=off  SenseContactBaseRotation=off  SenseContactBaseTranslation=off  SenseContactFollowerRotation=off  SenseContactFollowerTranslation=off  ZeroCrossDetectContactStartAndEnd=off
  Transform Sensor : sm_lib/Frames and Transforms/Transform Sensor  MeasurementFrame=Base  RotationSequence=ZYX  SenseAngle=off  SenseAxis=off  SenseQ=off  SenseR=off  SenseRotationSequence=on  SenseOmegaX=off  SenseOmegaY=off  SenseOmegaZ=off  SenseOmega=off  SenseQDot=off  SenseRDot=off  SenseRotationSequenceDot=off  SenseAlphaX=off  SenseAlphaY=off  SenseAlphaZ=off  SenseAlpha=off  SenseQDDot=off  SenseRDDot=off  SenseX=off  SenseY=off  SenseZ=off  SenseXYZ=off  SenseRad=off  SenseAzim=off  SenseDist=off  SenseInc=off  SenseXDot=off  SenseYDot=off  SenseZDot=off  SenseXYZDot=off  SenseRadDot=off  SenseAzimDot=off  SenseDistDot=off  SenseIncDot=off  SenseXDDot=off  SenseYDDot=off  SenseZDDot=off  SenseXYZDDot=off  SenseRadDDot=off  SenseAzimDDot=off  SenseDistDDot=off  SenseIncDDot=off
  World Frame : sm_lib/Frames and Transforms/World Frame
  Main Body Data : Outport
  Left Motor1 Data : Outport  Port=2
  Left Motor2 Data : Outport  Port=3
  Right Motor2 Data : Outport  Port=4
  Right Motor1 Data : Outport  Port=5
  Left Wheel Data : Outport  Port=6
  Right  Wheel Data : Outport  Port=7
  wires:
  PS-Simulink Converter6/1 -> Bus Creator/7  "pos z"
  PS-Simulink Converter1/1 -> Bus Creator/2  "vel x"
  PS-Simulink Converter2/1 -> Bus Creator/3  "acc x"
  PS-Simulink Converter4/1 -> Bus Creator/5  "vel y"
  PS-Simulink Converter5/1 -> Bus Creator/6  "acc y"
  PS-Simulink Converter3/1 -> Bus Creator/4  "pos y"
  PS-Simulink Converter8/1 -> Bus Creator/9  "acc z"
  PS-Simulink Converter7/1 -> Bus Creator/8  "vel z"
  PS-Simulink Converter/1 -> Bus Creator/1  "pos x"
  Bus Creator/1 -> Main Body Data/1
  Left Motor1  Torque/1 -> Simulink-PS Converter/1
  Left Motor2 Torque/1 -> Simulink-PS Converter1/1
  RIght Motor2 Torque/1 -> Simulink-PS Converter2/1  "2"
  Right Wheel Torque/1 -> Simulink-PS Converter4/1
  Left Wheel Torque/1 -> Simulink-PS Converter5/1
  PS-Simulink Converter15/1 -> Bus Creator1/1  "angle"
  PS-Simulink Converter16/1 -> Bus Creator1/2  "velocity"
  PS-Simulink Converter17/1 -> Bus Creator1/3  "accel"
  PS-Simulink Converter18/1 -> Bus Creator1/4  "torque"
  Bus Creator1/1 -> Left Motor1 Data/1
  PS-Simulink Converter21/1 -> Bus Creator2/3  "accel"
  Bus Creator2/1 -> Left Motor2 Data/1
  PS-Simulink Converter20/1 -> Bus Creator2/2  "velocity"
  PS-Simulink Converter19/1 -> Bus Creator2/1  "angle"
  PS-Simulink Converter22/1 -> Bus Creator2/4  "torque"
  PS-Simulink Converter25/1 -> Bus Creator3/3  "accel"
  Bus Creator3/1 -> Right Motor2 Data/1
  PS-Simulink Converter24/1 -> Bus Creator3/2  "velocity"
  PS-Simulink Converter23/1 -> Bus Creator3/1  "angle"
  PS-Simulink Converter26/1 -> Bus Creator3/4  "torque"
  PS-Simulink Converter29/1 -> Bus Creator4/3  "accel"
  Bus Creator4/1 -> Right Motor1 Data/1
  PS-Simulink Converter28/1 -> Bus Creator4/2  "velocity"
  PS-Simulink Converter27/1 -> Bus Creator4/1  "angle"
  PS-Simulink Converter30/1 -> Bus Creator4/4  "torque"
  PS-Simulink Converter37/1 -> Bus Creator6/3  "accel"
  Bus Creator6/1 -> Left Wheel Data/1
  PS-Simulink Converter36/1 -> Bus Creator6/2  "velocity"
  PS-Simulink Converter35/1 -> Bus Creator6/1  "angle"
  PS-Simulink Converter38/1 -> Bus Creator6/4  "torque"
  PS-Simulink Converter34/1 -> Bus Creator5/4  "torque"
  PS-Simulink Converter31/1 -> Bus Creator5/1  "angle"
  PS-Simulink Converter32/1 -> Bus Creator5/2  "velocity"
  Bus Creator5/1 -> Right  Wheel Data/1
  PS-Simulink Converter33/1 -> Bus Creator5/3  "accel"
  Right Motor1 Torque/1 -> Simulink-PS Converter3/1  "1"
  PS-Simulink Converter11/1 -> Bus Creator/12  "acc yaw"
  PS-Simulink Converter10/1 -> Bus Creator/11  "acc pitch"
  PS-Simulink Converter9/1 -> Bus Creator/10  "acc roll"
  PS-Simulink Converter12/1 -> Demux/1  "ang"
  Demux/1 -> Bus Creator/13  "ang yaw"
  Demux/2 -> Bus Creator/14  "ang pitch"
  Demux/3 -> Bus Creator/15  "ang roll"
  connections:
  Initial height/LConn1 -- Solver Configuration/RConn1 -- Mechanism Configuration/RConn1 -- World Frame/RConn1 -- Ground/RConn1
  6-DOF Joint/RConn5 -- PS-Simulink Converter3/LConn1
  6-DOF Joint/RConn12 -- PS-Simulink Converter10/LConn1
  6-DOF Joint/RConn8 -- PS-Simulink Converter6/LConn1
  6-DOF Joint/RConn3 -- PS-Simulink Converter1/LConn1
  6-DOF Joint/RConn6 -- PS-Simulink Converter4/LConn1
  Initial height/RConn1 -- Transform Sensor/LConn1 -- 6-DOF Joint/LConn1
  6-DOF Joint/RConn4 -- PS-Simulink Converter2/LConn1
  6-DOF Joint/RConn2 -- PS-Simulink Converter/LConn1
  6-DOF Joint/RConn11 -- PS-Simulink Converter9/LConn1
  Ground/LConn1 -- Spatial Contact Force11/LConn1 -- Spatial Contact Force10/LConn1 -- Spatial Contact Force6/LConn1 -- Spatial Contact Force7/LConn1 -- Spatial Contact Force8/LConn1 -- Spatial Contact Force9/LConn1 -- Spatial Contact Force5/LConn1 -- Spatial Contact Force4/LConn1 -- Spatial Contact Force3/LConn1 -- Spatial Contact Force2/LConn1 -- Spatial Contact Force1/LConn1 -- Spatial Contact Force/LConn1
  6-DOF Joint/RConn7 -- PS-Simulink Converter5/LConn1
  6-DOF Joint/RConn9 -- PS-Simulink Converter7/LConn1
  6-DOF Joint/RConn13 -- PS-Simulink Converter11/LConn1
  6-DOF Joint/RConn10 -- PS-Simulink Converter8/LConn1
  Spatial Contact Force/RConn1 -- Main Body/LConn2
  Load/RConn1 -- Transform Sensor/RConn1 -- 6-DOF Joint/RConn1 -- Main Body/LConn1
  Spatial Contact Force1/RConn1 -- Load/LConn1
  Main Body/RConn1 -- Rigid Transform/LConn1
  Rigid Transform/RConn1 -- Left Motor1/LConn1
  Left Motor2/LConn1 -- Rigid Transform1/RConn1
  Main Body/RConn2 -- Rigid Transform1/LConn1
  Main Body/RConn3 -- Rigid Transform2/LConn1
  Right Motor2/LConn1 -- Rigid Transform2/RConn1
  Right Motor1/LConn1 -- Rigid Transform3/RConn1
  Main Body/RConn4 -- Rigid Transform3/LConn1
  Left Motor1/RConn1 -- Left Big Rod1/LConn2
  Left Motor2/RConn1 -- Left Big Rod2/LConn2
  Right Motor2/RConn1 -- Right Big Rod2/LConn2
  Right Motor1/RConn1 -- Right Big Rod1/LConn2
  Left Little Rod1/LConn2 -- Left Big Rod1/RConn1
  Left Little Rod2/LConn2 -- Left Big Rod2/RConn1
  Revolute Joint/LConn1 -- Left Little Rod2/RConn1 -- Left Wheel/LConn1
  Left Little Rod1/RConn1 -- Revolute Joint/RConn1
  Right Little Rod2/RConn1 -- Revolute Joint1/RConn1
  Right Wheel/LConn1 -- Rigid Transform4/RConn1
  Right Little Rod1/LConn2 -- Right Big Rod1/RConn1
  Right Little Rod2/LConn2 -- Right Big Rod2/RConn1
  Spatial Contact Force3/RConn1 -- Left Big Rod2/LConn1
  Left Big Rod1/LConn1 -- Spatial Contact Force2/RConn1
  Spatial Contact Force4/RConn1 -- Right Big Rod2/LConn1
  Right Big Rod1/LConn1 -- Spatial Contact Force5/RConn1
  Spatial Contact Force8/RConn1 -- Left Little Rod2/LConn1
  Spatial Contact Force7/RConn1 -- Right Little Rod2/LConn1
  Spatial Contact Force6/RConn1 -- Right Little Rod1/LConn1
  Left Little Rod1/LConn1 -- Spatial Contact Force9/RConn1
  Left Wheel/LConn3 -- Spatial Contact Force10/RConn1
  Right Wheel/LConn3 -- Spatial Contact Force11/RConn1
  Simulink-PS Converter/RConn1 -- Left Motor1/LConn2
  Left Motor2/LConn2 -- Simulink-PS Converter1/RConn1
  Right Wheel/LConn2 -- Simulink-PS Converter4/RConn1
  Simulink-PS Converter5/RConn1 -- Left Wheel/LConn2
  PS-Simulink Converter15/LConn1 -- Left Motor1/RConn2
  PS-Simulink Converter16/LConn1 -- Left Motor1/RConn3
  Left Motor1/RConn4 -- PS-Simulink Converter17/LConn1
  Left Motor1/RConn5 -- PS-Simulink Converter18/LConn1
  Left Motor2/RConn2 -- PS-Simulink Converter19/LConn1
  Left Motor2/RConn3 -- PS-Simulink Converter20/LConn1
  Left Motor2/RConn5 -- PS-Simulink Converter22/LConn1
  Left Motor2/RConn4 -- PS-Simulink Converter21/LConn1
  Right Motor2/RConn2 -- PS-Simulink Converter23/LConn1
  PS-Simulink Converter24/LConn1 -- Right Motor2/RConn3
  Right Motor2/RConn5 -- PS-Simulink Converter26/LConn1
  PS-Simulink Converter25/LConn1 -- Right Motor2/RConn4
  Right Motor1/RConn2 -- PS-Simulink Converter27/LConn1
  Right Motor1/RConn3 -- PS-Simulink Converter28/LConn1
  Right Motor1/RConn5 -- PS-Simulink Converter30/LConn1
  Right Motor1/RConn4 -- PS-Simulink Converter29/LConn1
  Left Wheel/RConn1 -- PS-Simulink Converter35/LConn1
  Left Wheel/RConn2 -- PS-Simulink Converter36/LConn1
  Left Wheel/RConn4 -- PS-Simulink Converter38/LConn1
  Left Wheel/RConn3 -- PS-Simulink Converter37/LConn1
  Right Wheel/RConn1 -- PS-Simulink Converter31/LConn1
  Right Wheel/RConn2 -- PS-Simulink Converter32/LConn1
  Right Wheel/RConn3 -- PS-Simulink Converter33/LConn1
  Right Wheel/RConn4 -- PS-Simulink Converter34/LConn1
  Rigid Transform4/LConn1 -- Revolute Joint1/LConn1 -- Right Little Rod1/RConn1
  Simulink-PS Converter2/RConn1 -- Right Motor2/LConn2
  Simulink-PS Converter3/RConn1 -- Right Motor1/LConn2
  PS-Simulink Converter12/LConn1 -- Transform Sensor/RConn2

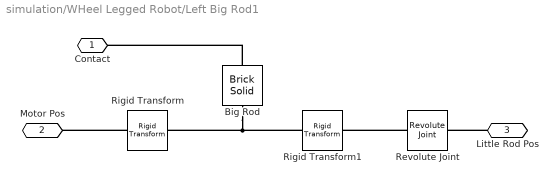
== system simulation/WHeel Legged Robot/Left Big Rod1 ==
  Big Rod : sm_lib/Body Elements/Brick Solid  BrickDimensions=[BR_L BR_W BR_H]  BrickDimensionsUnits=mm  ExportEntireGeometry=on  InertiaType=CalculateFromGeometry  BasedOnType=Mass  Density=1000  DensityUnits=kg/m^3  Mass=BR_M  MassUnits=kg  CenterOfMass=[0 0 0]  CenterOfMassUnits=m  MomentsOfInertia=[1 1 1]  MomentsOfInertiaUnits=kg*m^2  ProductsOfInertia=[0 0 0]  ProductsOfInertiaUnits=kg*m^2  GraphicType=FromGeometry  MarkerShape=Sphere  MarkerSize=10  GraphicVisPropType=SimpleVisualProperties  GraphicDiffuseColor=[1 0.7333 0]  GraphicOpacity=1  GraphicSpecularColor=[0.5 0.5 0.5 1.0]  GraphicAmbientColor=[0.15 0.15 0.15 1.0]  GraphicEmissiveColor=[0.0 0.0 0.0 1.0]  GraphicShininess=75  DoExposeReferenceFrame=on  SerializedFrames=<Frames/>
  Revolute Joint : sm_lib/Joints/Revolute Joint  JointMode=Normal  CompositeWrenchDir=FollowerOnBase  CompositeWrenchFrame=BaseFrame  SenseConstraintForce=off  SenseConstraintTorque=off  SenseTotalForce=off  SenseTotalTorque=off  PositionTargetSpecify=off  PositionTargetPriority=High  PositionTargetValue=0  PositionTargetValueUnits=deg  VelocityTargetSpecify=off  VelocityTargetPriority=High  VelocityTargetValue=0  VelocityTargetValueUnits=deg/s  EquilibriumPosition=0  EquilibriumPositionUnits=deg  SpringStiffness=0  SpringStiffnessUnits=N*m/deg  DampingCoefficient=0  DampingCoefficientUnits=N*m/(deg/s)  LowerLimitSpecify=off  LowerLimitBound=JO_Min_A  LowerLimitBoundUnits=deg  LowerLimitStiffness=1e4  LowerLimitStiffnessUnits=N*m/deg  LowerLimitDamping=10  LowerLimitDampingUnits=N*m/(deg/s)  LowerLimitTransitionRegionWidth=0.1  LowerLimitTransitionRegionWidthUnits=deg  UpperLimitSpecify=off  UpperLimitBound=JO_Max_A  UpperLimitBoundUnits=deg  UpperLimitStiffness=1e4  UpperLimitStiffnessUnits=N*m/deg  UpperLimitDamping=10  UpperLimitDampingUnits=N*m/(deg/s)  UpperLimitTransitionRegionWidth=0.1  UpperLimitTransitionRegionWidthUnits=deg  TorqueActuationMode=NoTorque  MotionActuationMode=ComputedMotion  SensePosition=off  SenseVelocity=off  SenseAcceleration=off  SenseTorqueForce=off  SenseLowerLimitTorqueForce=off  SenseUpperLimitTorqueForce=off
  Rigid Transform : sm_lib/Frames and Transforms/Rigid Transform  RotationMethod=None  FollAlignAxisA=+X  BaseAlignAxisA=+Y  FollAlignAxisB=+Y  BaseAlignAxisB=+Z  RotationStandardAxis=+Z  RotationAngle=0  RotationAngleUnits=deg  RotationArbitraryAxis=[0 0 1]  RotationSequenceAxes=FollowerAxes  RotationSequence=XYX  RotationSequenceAngles=[0 0 0]  RotationSequenceAnglesUnits=deg  RotationMatrix=[1 0 0;0 1 0;0 0 1]  Quaternion=[1 0 0 0]  TranslationMethod=StandardAxis  TranslationCartesianOffset=[0 0 0]  TranslationCartesianOffsetUnits=m  TranslationStandardAxis=-X  TranslationStandardOffset=BR_L/2  TranslationStandardOffsetUnits=mm  TranslationROffset=0  TranslationROffsetUnits=m  TranslationThetaOffset=0  TranslationThetaOffsetUnits=deg  TranslationZOffset=0  TranslationZOffsetUnits=m
  Rigid Transform1 : sm_lib/Frames and Transforms/Rigid Transform  RotationMethod=None  FollAlignAxisA=+X  BaseAlignAxisA=+Y  FollAlignAxisB=+Y  BaseAlignAxisB=+Z  RotationStandardAxis=+Z  RotationAngle=0  RotationAngleUnits=deg  RotationArbitraryAxis=[0 0 1]  RotationSequenceAxes=FollowerAxes  RotationSequence=XYX  RotationSequenceAngles=[0 0 0]  RotationSequenceAnglesUnits=deg  RotationMatrix=[1 0 0;0 1 0;0 0 1]  Quaternion=[1 0 0 0]  TranslationMethod=StandardAxis  TranslationCartesianOffset=[0 0 0]  TranslationCartesianOffsetUnits=m  TranslationStandardAxis=+X  TranslationStandardOffset=BR_L/2  TranslationStandardOffsetUnits=mm  TranslationROffset=0  TranslationROffsetUnits=m  TranslationThetaOffset=0  TranslationThetaOffsetUnits=deg  TranslationZOffset=0  TranslationZOffsetUnits=m
  Contact : PMIOPort  Side=Left
  Motor Pos : PMIOPort  Port=2  Side=Left
  Little Rod Pos : PMIOPort  Port=3  Side=Right
  connections:
  Big Rod/LConn1 -- Contact/RConn1
  Big Rod/RConn1 -- Rigid Transform/LConn1 -- Rigid Transform1/LConn1
  Rigid Transform/RConn1 -- Motor Pos/RConn1
  Revolute Joint/LConn1 -- Rigid Transform1/RConn1
  Little Rod Pos/RConn1 -- Revolute Joint/RConn1
